simulink library "command_processing"  (R2016b)
settings: Solver=VariableStepAuto  StartTime=0.0  StopTime=10.0  RelTol=1e-3
undefined symbols (not defined in the file or in its folder): DiscIntNeverNeededParam, fsw_params
libraries: aerolibutil x1
settings Model: Creator=taylorreynolds  LastModifiedBy=Taylor

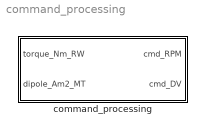
== system command_processing ==
  command_processing : Subsystem

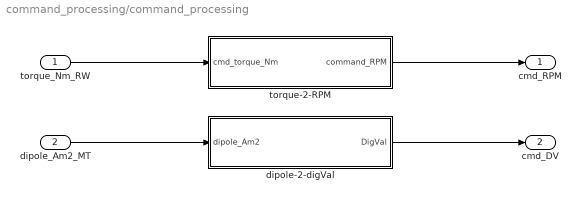
== system command_processing/command_processing ==
  torque_Nm_RW : Inport
  dipole_Am2_MT : Inport  Port=2
  dipole-2-digVal : Subsystem
  torque-2-RPM : Subsystem
  cmd_RPM : Outport
  cmd_DV : Outport  Port=2
  wires:
  torque-2-RPM/1(command_RPM) -> cmd_RPM/1
  torque_Nm_RW/1 -> torque-2-RPM/1(cmd_torque_Nm)
  dipole_Am2_MT/1 -> dipole-2-digVal/1(dipole_Am2)
  dipole-2-digVal/1(DigVal) -> cmd_DV/1

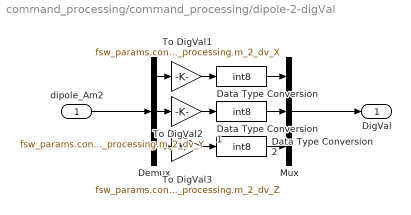
== system command_processing/command_processing/dipole-2-digVal ==
  dipole_Am2 : Inport
  Data Type Conversion : DataTypeConversion  OutDataTypeStr=int8  RndMeth=Nearest
  Data Type Conversion1 : DataTypeConversion  OutDataTypeStr=int8  RndMeth=Nearest
  Data Type Conversion2 : DataTypeConversion  OutDataTypeStr=int8  RndMeth=Nearest
  Demux : Demux  Outputs=3
  Mux : Mux  Inputs=3
  To DigVal1 : Gain  Gain=fsw_params.control.cmd_processing.m_2_dv_X
  To DigVal2 : Gain  Gain=fsw_params.control.cmd_processing.m_2_dv_Y
  To DigVal3 : Gain  Gain=fsw_params.control.cmd_processing.m_2_dv_Z
  DigVal : Outport
  wires:
  dipole_Am2/1 -> Demux/1
  Demux/3 -> To DigVal3/1
  Demux/2 -> To DigVal2/1
  Demux/1 -> To DigVal1/1
  To DigVal1/1 -> Data Type Conversion/1
  To DigVal2/1 -> Data Type Conversion1/1
  To DigVal3/1 -> Data Type Conversion2/1
  Mux/1 -> DigVal/1
  Data Type Conversion/1 -> Mux/1
  Data Type Conversion1/1 -> Mux/2
  Data Type Conversion2/1 -> Mux/3

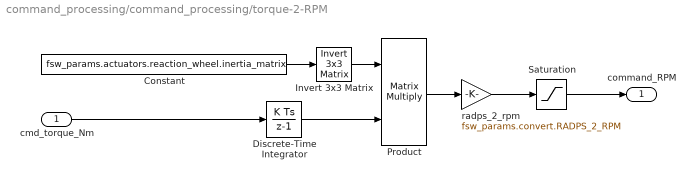
== system command_processing/command_processing/torque-2-RPM ==
  cmd_torque_Nm : Inport
  Constant : Constant  Value=fsw_params.actuators.reaction_wheel.inertia_matrix
  Discrete-Time Integrator : DiscreteIntegrator  InitialCondition=fsw_params.control.cmd_processing.ic.torque  InitialConditionSetting=State (most efficient)  SampleTime=-1  ICPrevOutput=DiscIntNeverNeededParam  ICPrevScaledInput=DiscIntNeverNeededParam
  Invert 3x3 Matrix : aerolibutil/Invert  3x3 Matrix
  Product : Product  Multiplication=Matrix(*)
  Saturation : Saturate  UpperLimit=fsw_params.actuators.reaction_wheel.max_RPM  LowerLimit=-fsw_params.actuators.reaction_wheel.max_RPM
  radps_2_rpm : Gain  Gain=fsw_params.convert.RADPS_2_RPM
  command_RPM : Outport
  wires:
  Constant/1 -> Invert 3x3 Matrix/1
  Invert 3x3 Matrix/1 -> Product/1
  Product/1 -> radps_2_rpm/1
  radps_2_rpm/1 -> Saturation/1
  cmd_torque_Nm/1 -> Discrete-Time Integrator/1
  Discrete-Time Integrator/1 -> Product/2
  Saturation/1 -> command_RPM/1
